simulink subsystem "Motors"  (R2024a)
settings: Solver=VariableStepAuto  StartTime=0.0  StopTime=10.0  RelTol=1e-3
libraries: stm32l4xxblockslib x2, stm32f4xxblockslib x1
settings Model: Creator=JesseJabezArendse  LastModifiedBy=emanu
settings RTWCC: GPUComputeCapability=3.5

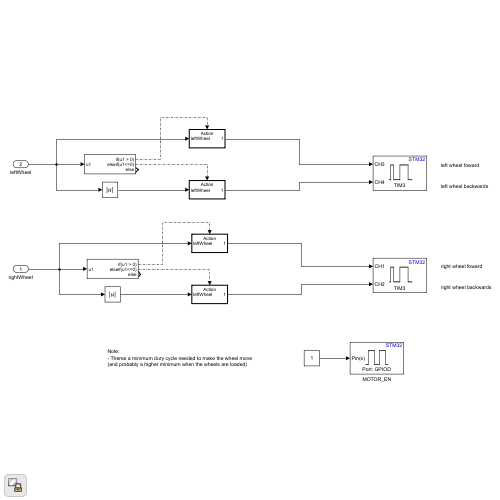
[thumbnail: Simulink's stored preview of the top-level diagram]
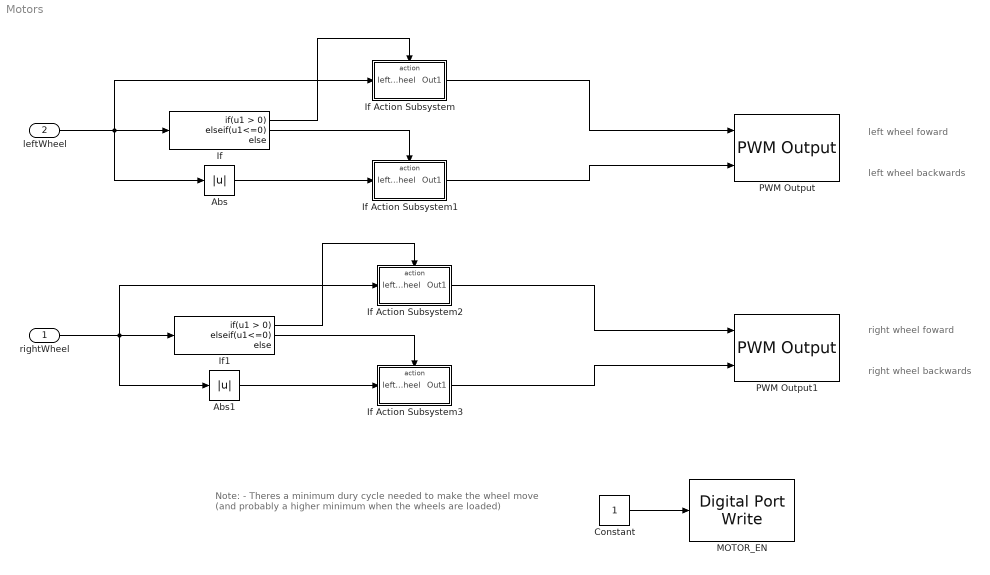
== system Motors ==
  note: Note:
      | - Theres a minimum dury cycle needed to make the wheel move (and probably a higher minimum when the wheels are loaded)
  note: left wheel foward
  note: left wheel backwards
  note: right wheel backwards
  note: right wheel foward
  rightWheel : Inport
  leftWheel : Inport  Port=2
  Abs : Abs  SaturateOnIntegerOverflow=off
  Abs1 : Abs  SaturateOnIntegerOverflow=off
  Constant : Constant
  If : If  ElseIfExpressions=u1<=0
  If Action Subsystem : Subsystem  TreatAsAtomicUnit=on
  If Action Subsystem1 : Subsystem  TreatAsAtomicUnit=on
  If Action Subsystem2 : Subsystem  TreatAsAtomicUnit=on
  If Action Subsystem3 : Subsystem  TreatAsAtomicUnit=on
  If1 : If  ElseIfExpressions=u1<=0
  MOTOR_EN : stm32f4xxblockslib/Digital Port Write  PortName=GPIOD  PinNumber=7  ReadOperation=off  IOAsArray=on  EnableSimPort=off  hoistedMaskSrc=ECSoC/ECSimCodegen/Digital Port Write
      settings: LibrarySourceBlock=stm32l4xxblockslib/Digital Port Write
  PWM Output : stm32l4xxblockslib/PWM Output  TimerModule=TIM3  DutycycleUnits=Percentage  EnableChannel1=off  EnableChannel2=off  EnableChannel3=on  EnableChannel4=on  EnableChannel5=off  EnableChannel6=off  EnableCounterInput=off  EnableMainOutputInput=off  EnableFrequencyInput=off  SetRCAfterCE=off  OutputDirection=off  OutputMainOutputEnableStatus=off  SampleTime=0.1  EnableSimPort=off  EnableUpdateEvent=off  EnableCaptureCompare1Event=off  EnableCaptureCompare2Event=off  EnableCaptureCompare3Event=off  EnableCaptureCompare4Event=off  EnableTriggerEvent=off  EnableBreakEvent=off  EnableBreakEvent2=off  ProcessorFamily=STM32L4  hoistedMaskSrc=ECSoC/ECSimCodegen/PWM Output
  PWM Output1 : stm32l4xxblockslib/PWM Output  TimerModule=TIM3  DutycycleUnits=Percentage  EnableChannel1=on  EnableChannel2=on  EnableChannel3=off  EnableChannel4=off  EnableChannel5=off  EnableChannel6=off  EnableCounterInput=off  EnableMainOutputInput=off  EnableFrequencyInput=off  SetRCAfterCE=off  OutputDirection=off  OutputMainOutputEnableStatus=off  SampleTime=0.1  EnableSimPort=off  EnableUpdateEvent=off  EnableCaptureCompare1Event=off  EnableCaptureCompare2Event=off  EnableCaptureCompare3Event=off  EnableCaptureCompare4Event=off  EnableTriggerEvent=off  EnableBreakEvent=off  EnableBreakEvent2=off  ProcessorFamily=STM32L4  hoistedMaskSrc=ECSoC/ECSimCodegen/PWM Output
  wires:
  Constant/1 -> MOTOR_EN/1
  leftWheel/1 -> If Action Subsystem/1(leftWheel), Abs/1, If/1
  If/1 -> If Action Subsystem/Action
  Abs/1 -> If Action Subsystem1/1(leftWheel)
  If Action Subsystem/1(Out1) -> PWM Output/1
  If Action Subsystem1/1(Out1) -> PWM Output/2
  If/2 -> If Action Subsystem1/Action
  If1/1 -> If Action Subsystem2/Action
  rightWheel/1 -> If Action Subsystem2/1(leftWheel), Abs1/1, If1/1
  If Action Subsystem3/1(Out1) -> PWM Output1/2
  If Action Subsystem2/1(Out1) -> PWM Output1/1
  If1/2 -> If Action Subsystem3/Action
  Abs1/1 -> If Action Subsystem3/1(leftWheel)

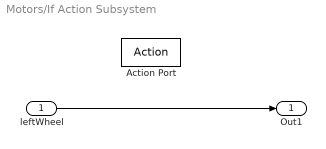
== system Motors/If Action Subsystem ==
  leftWheel : Inport
  Action Port : ActionPort
  Out1 : Outport  OutputWhenDisabled=reset  InitialOutput=0
  wires:
  leftWheel/1 -> Out1/1

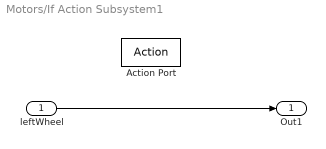
== system Motors/If Action Subsystem1 ==
  leftWheel : Inport
  Action Port : ActionPort
  Out1 : Outport  OutputWhenDisabled=reset  InitialOutput=0
  wires:
  leftWheel/1 -> Out1/1

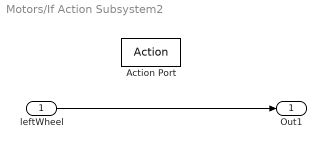
== system Motors/If Action Subsystem2 ==
  leftWheel : Inport
  Action Port : ActionPort
  Out1 : Outport  OutputWhenDisabled=reset  InitialOutput=0
  wires:
  leftWheel/1 -> Out1/1

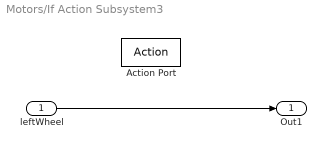
== system Motors/If Action Subsystem3 ==
  leftWheel : Inport
  Action Port : ActionPort
  Out1 : Outport  OutputWhenDisabled=reset  InitialOutput=0
  wires:
  leftWheel/1 -> Out1/1
